simulink model "limAzioneDerivativa"  (R2019a)
settings: Solver=VariableStepAuto  StartTime=0.0  StopTime=15  RelTol=1e-3
values from neighbouring files (symbols this model uses):
  b = 1    [mainLimAzioneDerivativa.m]
  c = 0    [mainLimAzioneDerivativa.m]
  Kd = 1    [mainLimAzioneDerivativa.m]
  Ki = 2    [mainAntiWindup1.m]    (also in mainAntiWindup2.m; mainBumpless.m; mainLimAzioneDerivativa.m = 1; mainWindupIntegrale.m)
  Kn = 1    [mainLimAzioneDerivativa.m]
  Kp = 2    [mainAntiWindup1.m]    (also in mainAntiWindup2.m; mainBumpless.m; mainLimAzioneDerivativa.m; mainWindupIntegrale.m = 0)
  N = 30    [mainLimAzioneDerivativa.m]
  Td = Kd/Kp    (= 0.5)    [mainLimAzioneDerivativa.m]
libraries: simulink x1
settings Model: Creator=adria  LastModifiedBy=adria

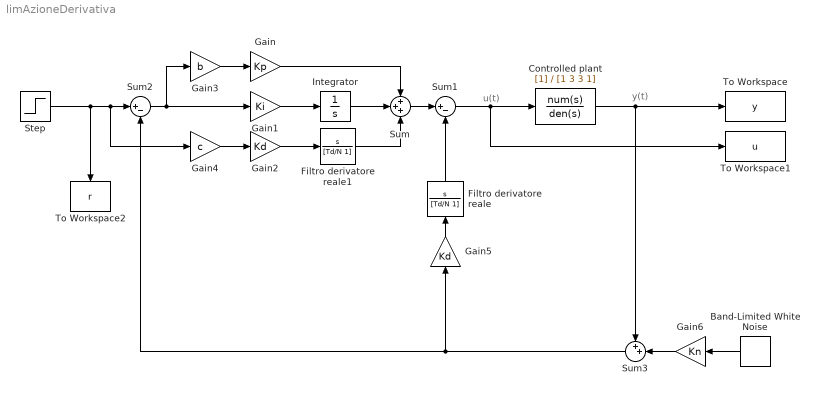
== system limAzioneDerivativa ==
  note: y(t)
  note: u(t)
  Band-Limited White Noise : simulink/Sources/Band-Limited White Noise  Cov=[0.01]  Ts=0.01  seed=[23341]
  Controlled plant : TransferFcn  Denominator=[1 3 3 1]
  Filtro derivatore reale : TransferFcn  Numerator=[1 0]  Denominator=[Td/N 1]
  Filtro derivatore reale1 : TransferFcn  Numerator=[1 0]  Denominator=[Td/N 1]
  Gain : Gain  Gain=Kp
  Gain1 : Gain  Gain=Ki
  Gain2 : Gain  Gain=Kd
  Gain3 : Gain  Gain=b
  Gain4 : Gain  Gain=c
  Gain5 : Gain  Gain=Kd
  Gain6 : Gain  Gain=Kn
  Integrator : Integrator
  Step : Step  SampleTime=0
  Sum : Sum  Inputs=+++
  Sum1 : Sum  Inputs=|+-
  Sum2 : Sum  Inputs=|+-
  Sum3 : Sum  Inputs=++|
  To Workspace : ToWorkspace  VariableName=y  SaveFormat=Structure With Time  SampleTime=-1
  To Workspace1 : ToWorkspace  VariableName=u  SaveFormat=Structure With Time  SampleTime=-1
  To Workspace2 : ToWorkspace  VariableName=r  SaveFormat=Structure With Time  SampleTime=-1
  wires:
  Gain3/1 -> Gain/1
  Gain4/1 -> Gain2/1
  Gain1/1 -> Integrator/1
  Integrator/1 -> Sum/2
  Gain/1 -> Sum/1
  Gain2/1 -> Filtro derivatore reale1/1
  Sum/1 -> Sum1/1
  Sum1/1 -> To Workspace1/1, Controlled plant/1
  Sum2/1 -> Gain3/1, Gain1/1
  Controlled plant/1 -> To Workspace/1, Sum3/1
  Step/1 -> To Workspace2/1, Gain4/1, Sum2/1
  Gain5/1 -> Filtro derivatore reale/1
  Filtro derivatore reale/1 -> Sum1/2
  Filtro derivatore reale1/1 -> Sum/3
  Band-Limited White Noise/1 -> Gain6/1
  Sum3/1 -> Sum2/2, Gain5/1
  Gain6/1 -> Sum3/2
